simulink model "animation"  (R2024b)
settings: Solver=FixedStepAuto  StartTime=0.0  StopTime=100  FixedStep=0.005  RelTol=1e-3
libraries: sim3dlib x12
settings Model: Creator=ander  LastModifiedBy=ander
settings DebuggingCC: AlgebraicLoopMsg=none

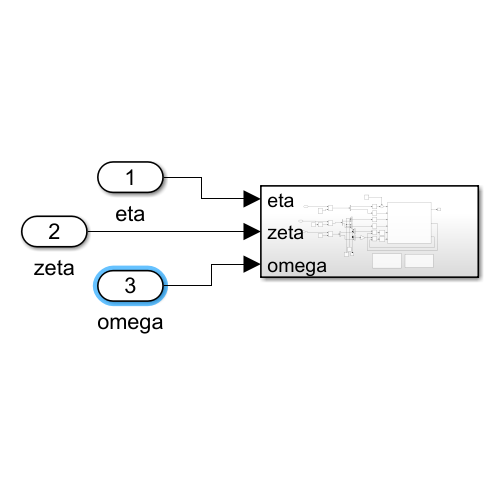
[thumbnail: Simulink's stored preview of the top-level diagram]
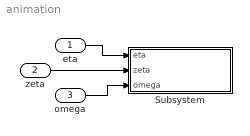
== system animation ==
  eta : Inport
  zeta : Inport  Port=2
  omega : Inport  Port=3
  Subsystem : Subsystem
  wires:
  zeta/1 -> Subsystem/2(zeta)
  omega/1 -> Subsystem/3(omega)
  eta/1 -> Subsystem/1(eta)

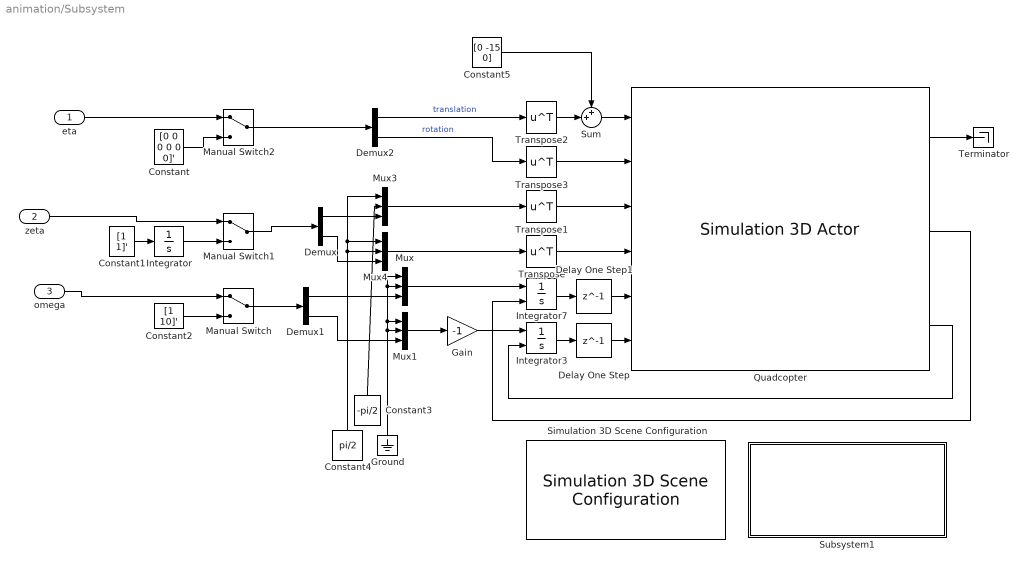
== system animation/Subsystem ==
  eta : Inport
  zeta : Inport  Port=2
  omega : Inport  Port=3
  Constant : Constant  Value=[0 0 0 0 0 0]'
  Constant1 : Constant  Value=[1 1]'
  Constant2 : Constant  Value=[1 10]'
  Constant3 : Constant  Value=-pi/2
  Constant4 : Constant  Value=pi/2
  Constant5 : Constant  Value=[0 -15 0]
  Delay One Step : Delay  DelayLength=1
  Delay One Step1 : Delay  DelayLength=1
  Demux : Demux  Outputs=2
  Demux1 : Demux  Outputs=2
  Demux2 : Demux  Outputs=2
  Gain : Gain  Gain=-1
  Ground : Ground
  Integrator : Integrator
  Integrator3 : Integrator  InitialConditionSource=external
  Integrator7 : Integrator  InitialConditionSource=external
  Manual Switch : ManualSwitch
  Manual Switch1 : ManualSwitch
  Manual Switch2 : ManualSwitch
  Mux{,1,3..4} (4 alike) : Mux  Inputs=3
  Quadcopter : sim3dlib/Simulation 3D Actor  ActorName=Quadcopter  ParentName=Scene Origin  Operation=Create at setup  InitScriptText=|  SampleTime=-1  Translation=single([-3.5 0 1.7])  Rotation=single([0 0 0])  Scale=single([1 1 1])  InputsText=|  OutputsText=BladeR.Rotation BladeL.Rotation  aMode=5  ActorTag=Quadcopter  ActorType=Sim3dActor  ID=C
      InitScriptText=|
      | fileNameBody = "bicopter/main.stl";
      | fileNameWing = "bicopter/wing simple.stl";
      | fileNameBlade = "bicopter/blade.stl";
      | 
      | wing_scale = 0.01;
      | 
      | % Body
      | Body = sim3d.Actor(ActorName='Body', ...
      |     Mobility=sim3d.utils.MobilityTypes.Movable);
      | add(World,Body,Actor);
      | 
      | load(Body,fileNameBody,[1 1 1]*0.1);
      | Body.Rotation = [-1/2*pi,0,pi];
      | Body.Translation = [2 0 1.0];
      | 
      | % Wings
      | WingR = sim3d.Actor(ActorName='WingR', ...
      |     Mobility=sim3d.utils.MobilityTypes.Movable);
      | add(World,WingR,Actor);
      | load(WingR, fileNameWing, [1 1 1]*wing_scale);
      | WingR.Rotation = [1/2*pi -1/2*pi 0];
      | WingR.Translation = [0.1 0.15-0.1 0.55];
      | WingR.Parent = Body;
      | 
      | 
      | WingL = sim3d.Actor(ActorName='WingL', ...
      |     Mobility=sim3d.utils.MobilityTypes.Movable);
      | add(World,WingL,Actor);
      | load(WingL, fileNameWing, [1 1 1]*wing_scale);
      | WingL.Rotation = [1/2*pi 1/2*pi 0];
      | WingL.Translation = [0.08 0.15-0.1 -0.37];
      | WingL.Parent = Body;
      | 
      | % Blades
      | BladeR = sim3d.Actor(ActorName='BladeR', ...
      |     Mobility=sim3d.utils.MobilityTypes.Movable);
      | add(World,BladeR,Actor);
      | load(BladeR, fileNameBlade,[1 1 1]*0.1);
      | BladeR.Rotation = [-1/2*pi 0 0];
      | BladeR.Translation = [0 0 0];
      | BladeR.Parent = WingR;
      | 
      | 
      | BladeL = sim3d.Actor(ActorName='BladeL', ...
      |     Mobility=sim3d.utils.MobilityTypes.Movable);
      | add(World,BladeL,Actor);
      | load(BladeL, fileNameBlade,[1 1 1]*0.1);
      | BladeL.Rotation = [-1/2*pi 0 0];
      | BladeL.Translation = [0 0 0];
      | BladeL.Parent = WingL;
      InputsText=|
      | Quadcopter.Translation
      | Quadcopter.Rotation
      | WingR.Rotation
      | WingL.Rotation
      | BladeR.Rotation
      | BladeL.Rotation
      settings: LibrarySourceBlock=sl3dlib/Simulation 3D/Simulation 3D Actor
  Simulation 3D Scene Configuration : sim3dlib/Simulation 3D Scene Configuration  Priority=0  ProjectFormat=Default Scenes  SceneDesc=Straight road  ProjectName=C:\Program Files\MATLAB\R2024b\toolbox\shared\sim3d_projects\automotive_project_windows\UE\WindowsNoEditor\VehicleSimulation.exe  ScenePath=/Game/Maps/HwStrght  EnableOpenDRIVE=off  vehTagList={'Quadcopter';'Scene Origin';'Sim3dActor10';'Sim3dActor11';'Sim3dActor12';'Sim3dActor13';'Sim3dActor2';'Sim3dActor3';'Sim3dActor4';'Sim3dActor5';'Sim3dActor6';'Sim3dActor7';'Sim3dActor8';'Sim3dActor9'}  vehTag=Quadcopter  FreeCameraInitialTranslation=[0, -15, 1]  FreeCameraDefaultInitialTranslation=[-6, 0, 2]  FreeCameraInitialRotation=[0, 0, 0]  FreeCameraDefaultInitialRotation=[0, -15, 0]  OpVisEn=off  Ts=.02  EnableWindow=on  EnableRemoteAccess=off  EnableWeather=off  SunAzimuth=90  SunAltitude=40.0  EnableGeospatialSun=off  Latitude=0  Longitude=0  Date=2023-01-01  Time=10:30:00  GeoTimeZone=-5.0  SunDaylightSaving=off  wind=1  clouds=10  EnableVolumetricClouds=off  CloudCoverage=0  CloudAltitude=6  fog=0  rain=0  RaindropsEffect=off  SnowDensity=85.0  EnableGeospatial=off  UseTrueOrigin=off  OriginHeight=200  OriginLatitude=40.744652  OriginLongitude=-73.988864  MapStyle=Aerial  AdditionalAssetIDs=[]  UseAdvancedSunSky=off  SolarTime=11  TimeZone=-5  Day=21  Month=9  Year=2022  UseDaylightSavingTime=on  DSTStartDay=10  DSTStartMonth=3  DSTEndDay=3  DSTEndMonth=11  DSTSwitchHour=2  sensorTag=MainCamera1  sensorId=1  sensorName=MainCamera1  mountLoc=Origin  offsetFlag=off  tmountOffset=[0, 0, 0]  rmountOffset=[0, 0, 0]  HorizontalResolution=1280  VerticalResolution=720  HorizontalFOV=60  mountPoint=[0 0 0]  mountOrientation=[0 0 0]  aMode=5  ID=1  GeoTrigger=Inactive
      settings: LibrarySourceBlock=sl3dlib/Simulation 3D/Environment/Simulation 3D Scene Configuration
  Subsystem1 : Subsystem
  Sum : Sum  Inputs=++|
  Terminator : Terminator
  Transpose{,1..3} (4 alike) : Math  Operator=transpose
  wires:
  Constant5/1 -> Sum/1
  Integrator/1 -> Manual Switch1/2
  omega/1 -> Manual Switch/1
  Delay One Step1/1 -> Quadcopter/5
  Demux2/2 -> Transpose3/1  "rotation"
  Mux/1 -> Integrator7/1
  Quadcopter/2 -> Integrator7/2
  eta/1 -> Manual Switch2/1
  Transpose1/1 -> Quadcopter/3
  Integrator3/1 -> Delay One Step/1
  Constant3/1 -> Mux3/2
  Ground/1 -> Mux/1, Mux/2, Mux1/1, Mux1/2
  Delay One Step/1 -> Quadcopter/6
  Transpose/1 -> Quadcopter/4
  Mux3/1 -> Transpose1/1
  Quadcopter/3 -> Integrator3/2
  zeta/1 -> Manual Switch1/1
  Mux4/1 -> Transpose/1
  Transpose2/1 -> Sum/2
  Quadcopter/1 -> Terminator/1
  Manual Switch2/1 -> Demux2/1
  Manual Switch/1 -> Demux1/1
  Constant1/1 -> Integrator/1
  Mux1/1 -> Gain/1
  Constant4/1 -> Mux3/1, Mux4/1, Mux4/2
  Demux2/1 -> Transpose2/1  "translation"
  Integrator7/1 -> Delay One Step1/1
  Demux1/1 -> Mux/3
  Gain/1 -> Integrator3/1
  Constant/1 -> Manual Switch2/2
  Demux1/2 -> Mux1/3
  Demux/2 -> Mux4/3
  Transpose3/1 -> Quadcopter/2
  Demux/1 -> Mux3/3
  Manual Switch1/1 -> Demux/1
  Constant2/1 -> Manual Switch/2
  Sum/1 -> Quadcopter/1

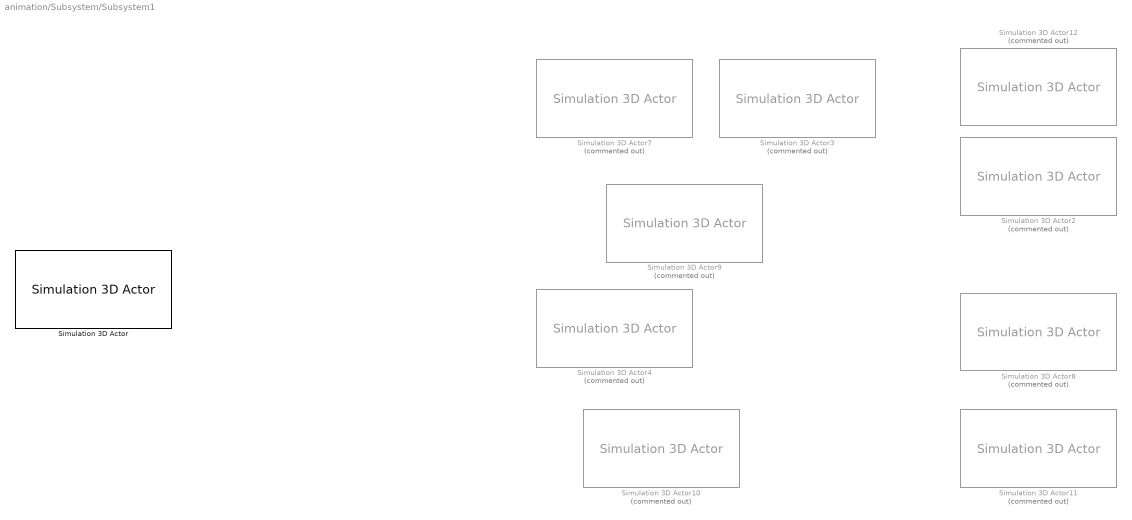
== system animation/Subsystem/Subsystem1 ==
  Simulation 3D Actor : sim3dlib/Simulation 3D Actor  Priority=1  ActorName=Sim3dActor14  ParentName=Scene Origin  Operation=Create at setup  InitScriptText=|  SampleTime=-1  Translation=[0 0 0]  Rotation=[0 0 0]  Scale=[1 1 1]  aMode=5  ActorTag=Sim3dActor14  ActorType=Sim3dActor  ID=14
      | createShape(Actor, 'box', [1 1 1]);
      | Actor.Color = [1 0 0];
  Simulation 3D Actor10 : sim3dlib/Simulation 3D Actor  Priority=1  Commented=on  ActorName=Sim3dActor15  ParentName=Scene Origin  Operation=Create at setup  InitScriptText=|  SampleTime=-1  Translation=[-20 -15 -0.5]  Rotation=[0 0 -1.5708]  Scale=[0.00375 0.00375 0.00375]  aMode=5  ActorTag=Sim3dActor15  ActorType=Sim3dActor  ID=15
      | fileName = "environment/fieldC.fbx";
      | 
      | posX = -20;
      | posY = -15;
      | posZ = -0.5;
      | 
      | scale = 0.005*0.75;
      | 
      | 
      | Body = sim3d.Actor(ActorName='Body', ...
      |     Mobility=sim3d.utils.MobilityTypes.Movable);
      | add(World,Body,Actor);
      | load(Body,fileName,[1 1 1]);
      | 
      | Actor.Rotation = [0 0 -pi/2];
      | Actor.Translation = [posX posY posZ];
      | Actor.Scale = [scale, scale, scale];
  Simulation 3D Actor11 : sim3dlib/Simulation 3D Actor  Priority=1  Commented=on  ActorName=Sim3dActor16  ParentName=Scene Origin  Operation=Create at setup  InitScriptText=|  SampleTime=-1  Translation=[-40 25 -0.5]  Rotation=[0 0 1.5708]  Scale=[0.00375 0.00375 0.00375]  aMode=5  ActorTag=Sim3dActor16  ActorType=Sim3dActor  ID=16
      | fileName = "environment/fieldC.fbx";
      | 
      | posX = -40;
      | posY = 25;
      | posZ = -0.5;
      | 
      | scale = 0.005*0.75;
      | 
      | 
      | Body = sim3d.Actor(ActorName='Body', ...
      |     Mobility=sim3d.utils.MobilityTypes.Movable);
      | add(World,Body,Actor);
      | load(Body,fileName,[1 1 1]);
      | 
      | Actor.Rotation = [0 0 pi/2];
      | Actor.Translation = [posX posY posZ];
      | Actor.Scale = [scale, scale, scale];
  Simulation 3D Actor12 : sim3dlib/Simulation 3D Actor  Priority=1  Commented=on  ActorName=Sim3dActor17  ParentName=Scene Origin  Operation=Create at setup  InitScriptText=|  SampleTime=-1  Translation=[30 30 -0.5]  Rotation=[0 0 1.5708]  Scale=[0.00375 0.00375 0.00375]  aMode=5  ActorTag=Sim3dActor17  ActorType=Sim3dActor  ID=17
      | fileName = "environment/fieldC.fbx";
      | 
      | posX = 30;
      | posY = 30;
      | posZ = -0.5;
      | 
      | scale = 0.005*0.75;
      | 
      | 
      | Body = sim3d.Actor(ActorName='Body', ...
      |     Mobility=sim3d.utils.MobilityTypes.Movable);
      | add(World,Body,Actor);
      | load(Body,fileName,[1 1 1]);
      | 
      | Actor.Rotation = [0 0 pi/2];
      | Actor.Translation = [posX posY posZ];
      | Actor.Scale = [scale, scale, scale];
  Simulation 3D Actor2 : sim3dlib/Simulation 3D Actor  Priority=1  Commented=on  ActorName=Sim3dActor18  ParentName=Scene Origin  Operation=Create at setup  InitScriptText=|  SampleTime=-1  Translation=[20 24 0]  Rotation=[0 0 -1.5708]  Scale=[0.005 0.005 0.005]  aMode=5  ActorTag=Sim3dActor18  ActorType=Sim3dActor  ID=18
      | fileName = "environment/TannerC.fbx";
      | 
      | posX = 20;
      | posY = 24;
      | posZ = 0;
      | 
      | scale = 0.005;
      | 
      | Body = sim3d.Actor(ActorName='Body', ...
      |     Mobility=sim3d.utils.MobilityTypes.Movable);
      | add(World,Body,Actor);
      | load(Body,fileName,[1 1 1]);
      | 
      | Actor.Translation = [posX posY posZ];
      | Actor.Scale = [scale, scale, scale];
  Simulation 3D Actor3 : sim3dlib/Simulation 3D Actor  Priority=1  Commented=on  ActorName=Sim3dActor19  ParentName=Scene Origin  Operation=Create at setup  InitScriptText=|  SampleTime=-1  Translation=[30 -20 0]  Rotation=[0 0 1.5708]  Scale=[0.005 0.005 0.005]  aMode=5  ActorTag=Sim3dActor19  ActorType=Sim3dActor  ID=19
      | fileName = "environment/ForgeC.fbx";
      | 
      | posX = 30;
      | posY = -20;
      | posZ = 0;
      | 
      | scale = 0.005;
      | 
      | 
      | Body = sim3d.Actor(ActorName='Body', ...
      |     Mobility=sim3d.utils.MobilityTypes.Movable);
      | add(World,Body,Actor);
      | load(Body,fileName,[1 1 1]);
      | 
      | Actor.Rotation = [0 0 pi/2];
      | Actor.Translation = [posX posY posZ];
      | Actor.Scale = [scale, scale, scale];
  Simulation 3D Actor4 : sim3dlib/Simulation 3D Actor  Priority=1  Commented=on  ActorName=Sim3dActor20  ParentName=Scene Origin  Operation=Create at setup  InitScriptText=|  SampleTime=-1  Translation=[15 0 0]  Rotation=[0 0 0]  Scale=[0.005 0.005 0.005]  aMode=5  ActorTag=Sim3dActor20  ActorType=Sim3dActor  ID=20
      | fileName = "environment/farmhCT.fbx";
      | 
      | posX = 15;
      | posY = 0;
      | posZ = 0;
      | 
      | scale = 0.005;
      | 
      | 
      | Body = sim3d.Actor(ActorName='Body', ...
      |     Mobility=sim3d.utils.MobilityTypes.Movable);
      | add(World,Body,Actor);
      | load(Body,fileName,[1 1 1]);
      | 
      | Actor.Translation = [posX posY posZ];
      | Actor.Scale = [scale, scale, scale];
  Simulation 3D Actor7 : sim3dlib/Simulation 3D Actor  Priority=1  Commented=on  ActorName=Sim3dActor21  ParentName=Scene Origin  Operation=Create at setup  InitScriptText=|  SampleTime=-1  Translation=[10 -40 0]  Rotation=[0 0 -1.5708]  Scale=[0.005 0.005 0.005]  aMode=5  ActorTag=Sim3dActor21  ActorType=Sim3dActor  ID=21
      | fileName = "environment/MillC.fbx";
      | 
      | posX = 10;
      | posY = -40;
      | posZ = 0;
      | 
      | scale = 0.005;
      | 
      | 
      | Body = sim3d.Actor(ActorName='Body', ...
      |     Mobility=sim3d.utils.MobilityTypes.Movable);
      | add(World,Body,Actor);
      | load(Body,fileName,[1 1 1]);
      | 
      | Actor.Translation = [posX posY posZ];
      | Actor.Scale = [scale, scale, scale];
      | Actor.Rotation = [0, 0, -pi/2];
  Simulation 3D Actor8 : sim3dlib/Simulation 3D Actor  Priority=1  Commented=on  ActorName=Sim3dActor22  ParentName=Scene Origin  Operation=Create at setup  InitScriptText=|  SampleTime=-1  Translation=[15 -5 0]  Rotation=[0 0 -1.5708]  Scale=[0.005 0.005 0.005]  aMode=5  ActorTag=Sim3dActor22  ActorType=Sim3dActor  ID=22
      | fileName = "environment/farmhCT.fbx";
      | 
      | posX = 15;
      | posY = -5;
      | posZ = 0;
      | 
      | scale = 0.005;
      | 
      | 
      | Body = sim3d.Actor(ActorName='Body', ...
      |     Mobility=sim3d.utils.MobilityTypes.Movable);
      | add(World,Body,Actor);
      | load(Body,fileName,[1 1 1]);
      | 
      | Actor.Rotation = [0 0 -pi/2];
      | Actor.Translation = [posX posY posZ];
      | Actor.Scale = [scale, scale, scale];
  Simulation 3D Actor9 : sim3dlib/Simulation 3D Actor  Priority=1  Commented=on  ActorName=Sim3dActor23  ParentName=Scene Origin  Operation=Create at setup  InitScriptText=|  SampleTime=-1  Translation=[25 -23 -0.5]  Rotation=[0 0 -1.5708]  Scale=[0.00375 0.00375 0.00375]  aMode=5  ActorTag=Sim3dActor23  ActorType=Sim3dActor  ID=23
      | fileName = "environment/fieldC.fbx";
      | 
      | posX = 25;
      | posY = -23;
      | posZ = -0.5;
      | 
      | scale = 0.005*0.75;
      | 
      | Body = sim3d.Actor(ActorName='Body', ...
      |     Mobility=sim3d.utils.MobilityTypes.Movable);
      | add(World,Body,Actor);
      | load(Body,fileName,[1 1 1]);
      | 
      | Actor.Rotation = [0 0 -pi/2];
      | Actor.Translation = [posX posY posZ];
      | Actor.Scale = [scale, scale, scale];
